simulink model "SegheriaSCADAdinamica"  (R2024b)
settings: Solver=FixedStepAuto  StartTime=0.0  StopTime=Tsim  FixedStep=dT  RelTol=1e-3
values from neighbouring files (symbols this model uses):
  b = t + 2*s    (= 3.6)    [ParametriSegheria.m]    (also in ParametriSegheriaDinamica.m)
  dT = 0.025    [ParametriSegheria.m]    (also in ParametriSegheriaDinamica.m)
  h_index = [70, 80, 90, 100]    [ParametriSegheria.m]    (also in ParametriSegheriaDinamica.m)
  J1 = 8*1e6    (= 8000000)    [ParametriSegheriaDinamica.m]
  J2 = 0.9*1e6    (= 900000)    [ParametriSegheriaDinamica.m]
  kc = [0 35 40 50 55 90]    [ParametriSegheria.m]    (also in ParametriSegheriaDinamica.m = [0, 25, 30, 35, 50, 70])
  Kt = 2    [ParametriSegheria.m]    (also in ParametriSegheriaDinamica.m = 10000)
  Kt2 = 5    [ParametriSegheria.m]    (also in ParametriSegheriaDinamica.m = 4500)
  l_index = [20, 30, 40, 50]    [ParametriSegheria.m]    (also in ParametriSegheriaDinamica.m)
  Lt = 4    [ParametriSegheria.m]    (also in ParametriSegheriaDinamica.m)
  Mag_D1 = [0 randi([220 500], 1, 40)]    [ParametriSegheria.m]    (also in ParametriSegheriaDinamica.m)
  Mag_D2 = [0 randi([220 500], 1, 40)]    [ParametriSegheria.m]    (also in ParametriSegheriaDinamica.m)
  Mag_D3 = [0 randi([220 500], 1, 40)]    [ParametriSegheria.m]    (also in ParametriSegheriaDinamica.m)
  Mag_legno1 = [0 randi([1 5], 1, 40)]    [ParametriSegheria.m]    (also in ParametriSegheriaDinamica.m)
  Mag_legno2 = [0 randi([1 5], 1, 40)]    [ParametriSegheria.m]    (also in ParametriSegheriaDinamica.m)
  Mag_legno3 = [0 randi([1 5], 1, 40)]    [ParametriSegheria.m]    (also in ParametriSegheriaDinamica.m)
  n_linee = 3    [ParametriSegheria.m]    (also in ParametriSegheriaDinamica.m)
  omega_ref1 = 50    [ParametriSegheriaDinamica.m]
  omega_ref2 = 3000*(2*pi/60)    (= 314.159265359)    [ParametriSegheriaDinamica.m]
  Rc = 200    [ParametriSegheria.m]    (also in ParametriSegheriaDinamica.m)
  rho = [0, 450, 520, 590, 710, 780]*1e-9    [ParametriSegheriaDinamica.m]
  Rs = 800    [ParametriSegheria.m]    (also in ParametriSegheriaDinamica.m)
  SR = Rs/Rm    (= 5.33333333333)    [ParametriSegheria.m]    (also in ParametriSegheriaDinamica.m)
  SR2 = Rc/Rm2    (= 4)    [ParametriSegheria.m]    (also in ParametriSegheriaDinamica.m)
  V_mean1 = 0.75    [ParametriSegheriaDinamica.m]
  V_mean23 = 1    [ParametriSegheriaDinamica.m]
undefined symbols (not defined in the file or in its folder): h_start_1, h_start_2, h_start_3, h_start_4, h_start_5, h_start_6, l_start_1, l_start_2, l_start_3, l_start_4, l_start_5, l_start_6
libraries: simulink x24, slpidlib x18
(part 4 of 4)

== matlab function SegheriaSCADAdinamica/Linea 2/MATLAB Function ==
  data: u input; y output
function y = fcn(u)

    persistent n_prec

    if isempty(n_prec)
        n_prec = 0;
    end

    y = u - n_prec;


    n_prec = u;

== matlab function SegheriaSCADAdinamica/Linea 2/MATLAB Function1 ==
  data: u input; y output
function y = fcn(u)

    persistent n_prec

    if isempty(n_prec)
        n_prec = 0;
    end

    y = u - n_prec;

    n_prec = u;

== matlab function SegheriaSCADAdinamica/Linea 2/MATLAB Function2 ==
  settings: updateMethod=DISCRETE
  data: lama_usurata input; y output; tronco_finito input
function y = fcn(lama_usurata, tronco_finito)
    
    persistent cambia_lama
    if isempty(cambia_lama)
        cambia_lama = 0;
    end

    if lama_usurata == 1
        cambia_lama = 1;
    end

    if tronco_finito == 1 && cambia_lama == 1
        y = cambia_lama;
        cambia_lama = 0;
    else
        y = 0;
    end

== matlab function SegheriaSCADAdinamica/Linea 2/MATLAB Function3 ==
  settings: updateMethod=DISCRETE
  data: u input; y output; t input
function y = f(u, t)
persistent t_start active

if isempty(active)
    active = false;
    t_start = 0;
end

if u == 1 && ~active
    t_start = t;
    active = true;
end

if active
    if (t - t_start) <= 180
        y = 0;
    else
        y = 1;
        active = false;
    end
else
    y = 1;
end

== matlab function SegheriaSCADAdinamica/Linea 2/Macchina 1/Dinamica Macchina 1/MATLAB Function3 ==
  data: w input; Fc output; vf input; kc input; Dt input; Rs parameter; b parameter
function Fc = Fcfun(w, vf, kc, Dt, Rs, b)

if w < 0.01
    Fc = 0;
else
    Fc = kc*b*vf*Dt/(w*Rs);
end

== matlab function SegheriaSCADAdinamica/Linea 2/Macchina 1/Logica Macchina 1/MATLAB Function ==
  data: u input; y output; Mag_legno parameter
function y = fcn(u, Mag_legno)
    persistent counter
    if isempty(counter)
        counter = 1;
    end

    if u == 1
        counter = counter + 1;
    end

    y = counter;
    
    if y > length(Mag_legno)-1
        y = 0;
    end

end

== matlab function SegheriaSCADAdinamica/Linea 3/MATLAB Function ==
  data: u input; y output
function y = fcn(u)

    persistent n_prec

    if isempty(n_prec)
        n_prec = 0;
    end

    y = u - n_prec;


    n_prec = u;

== matlab function SegheriaSCADAdinamica/Linea 3/MATLAB Function1 ==
  data: u input; y output
function y = fcn(u)

    persistent n_prec

    if isempty(n_prec)
        n_prec = 0;
    end

    y = u - n_prec;

    n_prec = u;

== matlab function SegheriaSCADAdinamica/Linea 3/MATLAB Function2 ==
  settings: updateMethod=DISCRETE
  data: lama_usurata input; y output; tronco_finito input
function y = fcn(lama_usurata, tronco_finito)
    
    persistent cambia_lama
    if isempty(cambia_lama)
        cambia_lama = 0;
    end

    if lama_usurata == 1
        cambia_lama = 1;
    end

    if tronco_finito == 1 && cambia_lama == 1
        y = cambia_lama;
        cambia_lama = 0;
    else
        y = 0;
    end

== matlab function SegheriaSCADAdinamica/Linea 3/MATLAB Function3 ==
  settings: updateMethod=DISCRETE
  data: u input; y output; t input
function y = f(u, t)
persistent t_start active

if isempty(active)
    active = false;
    t_start = 0;
end

if u == 1 && ~active
    t_start = t;
    active = true;
end

if active
    if (t - t_start) <= 180
        y = 0;
    else
        y = 1;
        active = false;
    end
else
    y = 1;
end

== matlab function SegheriaSCADAdinamica/Linea 3/Macchina 1/Dinamica Macchina 1/MATLAB Function3 ==
  data: w input; Fc output; vf input; kc input; Dt input; Rs parameter; b parameter
function Fc = Fcfun(w, vf, kc, Dt, Rs, b)

if w < 0.01
    Fc = 0;
else
    Fc = kc*b*vf*Dt/(w*Rs);
end

== matlab function SegheriaSCADAdinamica/Linea 1/Macchina 2/Dinamica Macchina 2/MATLAB Function3 ==
  data: w input; Fc output; vf input; kc input; ns input; h input; Rs parameter; b parameter
function Fc = Fcfun(w, vf, kc, ns, h, Rs, b)

if w < 0.01
    Fc = 0;
else
    Fc = ns*kc*b*vf*h/(w*Rs);
end

== matlab function SegheriaSCADAdinamica/Linea 3/Macchina 1/Logica Macchina 1/MATLAB Function ==
  data: u input; y output; Mag_legno parameter
function y = fcn(u, Mag_legno)
    persistent counter
    if isempty(counter)
        counter = 1;
    end

    if u == 1
        counter = counter + 1;
    end

    y = counter;
    
    if y > length(Mag_legno)-1
        y = 0;
    end

end

== matlab function SegheriaSCADAdinamica/Controllo Magazzino/MATLAB Function6 ==
  data: u input; idx output; h_index parameter
function idx = find_index(u, h_index)
%#codegen

v = h_index;

idx = -1; % valore default se non trovato

for i = 1:length(v)
    if u == v(i)
        idx = i;
        return;
    end
end

== matlab function SegheriaSCADAdinamica/Controllo Magazzino/MATLAB Function7 ==
  data: u input; idx output; h_index parameter
function idx = find_index(u, h_index)
%#codegen

v = h_index;

idx = -1; % valore default se non trovato

for i = 1:length(v)
    if u == v(i)
        idx = i;
        return;
    end
end

== matlab function SegheriaSCADAdinamica/Controllo Magazzino/MATLAB Function8 ==
  data: u input; idx output; h_index parameter
function idx = find_index(u, h_index)
%#codegen

v = h_index;

idx = -1; % valore default se non trovato

for i = 1:length(v)
    if u == v(i)
        idx = i;
        return;
    end
end

== matlab function SegheriaSCADAdinamica/Controllo Magazzino/MATLAB Function9 ==
  data: u input; idx output; h_index parameter
function idx = find_index(u, h_index)
%#codegen

v = h_index;

idx = -1; % valore default se non trovato

for i = 1:length(v)
    if u == v(i)
        idx = i;
        return;
    end
end

== matlab function SegheriaSCADAdinamica/Controllo Magazzino/MATLAB Function10 ==
  data: u input; idx output; l_index parameter
function idx = find_index(u, l_index)
%#codegen

v = l_index;

idx = -1; % valore default se non trovato

for i = 1:length(v)
    if u == v(i)
        idx = i;
        return;
    end
end

== matlab function SegheriaSCADAdinamica/Controllo Magazzino/MATLAB Function11 ==
  data: u input; idx output; l_index parameter
function idx = find_index(u, l_index)
%#codegen

v = l_index;

idx = -1; % valore default se non trovato

for i = 1:length(v)
    if u == v(i)
        idx = i;
        return;
    end
end

== matlab function SegheriaSCADAdinamica/Controllo Magazzino/MATLAB Function12 ==
  data: u input; idx output; l_index parameter
function idx = find_index(u, l_index)
%#codegen

v = l_index;

idx = -1; % valore default se non trovato

for i = 1:length(v)
    if u == v(i)
        idx = i;
        return;
    end
end

== matlab function SegheriaSCADAdinamica/Controllo Magazzino/MATLAB Function13 ==
  data: u input; idx output; l_index parameter
function idx = find_index(u, l_index)
%#codegen

v = l_index;

idx = -1; % valore default se non trovato

for i = 1:length(v)
    if u == v(i)
        idx = i;
        return;
    end
end

== matlab function SegheriaSCADAdinamica/Controllo Magazzino/MATLAB Function14 ==
  data: h_next output; Magazzino output; stop output; l_next output; h_idx input; target_matrice parameter; n_assi input; l_idx input
function [h_next, Magazzino, stop, l_next] = fcn(h_idx, target_matrice, n_assi, l_idx)

[n_rows, n_cols] = size(target_matrice);

h_next = zeros(1,length(h_idx));
l_next = zeros(1,length(l_idx));

persistent MagazzinoReale
persistent x_hat
persistent P


if isempty(MagazzinoReale)
    MagazzinoReale = zeros(n_rows, n_cols);
    x_hat = zeros(n_rows, n_cols);
    P = eye(n_rows*n_cols);
end

for i = 1:length(n_assi)

    % Output iniziali
    h_next(i) = h_idx(i);
    l_next(i) = l_idx(i);

    MagazzinoReale(h_idx(i), l_idx(i)) = MagazzinoReale(h_idx(i), l_idx(i)) + n_assi(i);

end
    
% MISURA RUMOROSA
sigma = 0.1;
y = MagazzinoReale + sigma*randn(size(MagazzinoReale));


% APPIATTISCO MATRICE
x_hat_vec = x_hat(:);
y_vec = y(:);
u = zeros(size(x_hat_vec));

% PREDICTION
Q = 0.01*eye(length(x_hat_vec));
x_pred = x_hat_vec + u;
P_pred = P + Q;

% UPDATE
R = 1*eye(length(x_hat_vec));
K = P_pred / (P_pred + R);
x_hat_vec = x_pred + K*(y_vec - x_pred);
P = (eye(size(K)) - K)*P_pred;

x_hat = reshape(x_hat_vec, n_rows, n_cols);


for i = 1:length(n_assi)
    if MagazzinoReale(h_idx(i), l_idx(i)) >= target_matrice(h_idx(i), l_idx(i))


        deficit = target_matrice - MagazzinoReale;

        best_cost = inf;
        best_h = h_idx(i);
        best_l = l_idx(i);

        for h = 1:n_rows
            for l = 1:n_cols

                if deficit(h,l) > 0

                    % Penalità cambio lama
                    cambio = (l ~= l_idx(i));

                    % Funzione costo
                    cost = -deficit(h,l) + 60*cambio;

                    if cost < best_cost
                        best_cost = cost;
                        best_h = h;
                        best_l = l;
                    end
                end

            end
        end

        if best_cost < inf
            h_next(i) = best_h;
            l_next(i) = best_l;
        end

    end
end

if MagazzinoReale >= target_matrice
    stop = 1;
else
    stop = 0;
end

Magazzino = MagazzinoReale;

== matlab function SegheriaSCADAdinamica/Linea 3/Macchina 1/Logica Macchina 1/MATLAB Function1 ==
  settings: updateMethod=DISCRETE
  data: spessore input; u input; spessore2 input; diametro input; y output; larg_asse output; thickness output; finito output; prior output; likelihood output; posterior output; larg_stim output
function [y, larg_asse, thickness, finito, prior, likelihood, posterior, larg_stim]= fcn(spessore, u, spessore2, diametro)
    persistent counter 
  
    thin_cut = 4;

    max_assi = floor((diametro-thin_cut*spessore2) / spessore);
    finito = 0;

    sigma_larg = 10;
    sigma_D = 10;

    if diametro > 0
        misure_D = diametro + sigma_D * randn();
    else
        misure_D = diametro;
    end

    maxD = 1000;
    larg_vec = 0:maxD;

    prior = zeros(size(larg_vec));
    likelihood = zeros(size(larg_vec));
    posterior = zeros(size(larg_vec));

    if isempty(counter)
        counter = 0;
    end

    % Conto assi tagliate
    if u == 1
        counter = counter + 1;
    end

    % Quando finisco tronco segnalo e azzero counter
    if counter > max_assi + thin_cut
        finito = 1;
        counter = 0;
    end

    % SISTEMARE INCERTEZZA: propagata da D in L
    if counter == 0
        larg_asse = 0;
        larg_asseD = 0;
        thickness = 0;
        sigma_largD = 0;
    elseif counter <= thin_cut/2
        distanza_bordo = counter * spessore2;
        larg_asse = sqrt((diametro)^2-(spessore2 + diametro - 2*distanza_bordo)^2);
        thickness = spessore2;
        % prior
        larg_asseD = sqrt(abs((misure_D)^2-(spessore2 + misure_D - 2*distanza_bordo)^2));
        sigma_largD = abs((2*distanza_bordo - spessore2)/sqrt((2*distanza_bordo - spessore2)*(-2*distanza_bordo + 2*diametro + spessore2)));
    elseif counter > max_assi + thin_cut/2
        distanza_bordo = max_assi*spessore + (counter-max_assi)*spessore2;
        larg_asse = sqrt((diametro)^2-(spessore2 + diametro - 2*distanza_bordo)^2);
        thickness = spessore2;
        % prior
        larg_asseD = sqrt(abs((misure_D)^2-(spessore2 + misure_D - 2*distanza_bordo)^2));
        sigma_largD = abs((2*distanza_bordo - spessore2)/sqrt((2*distanza_bordo - spessore2)*(-2*distanza_bordo + 2*diametro + spessore2)));
    else
        % Calcolo larghezza delle assi
        distanza_bordo = thin_cut/2 * spessore2 + (counter-thin_cut/2) * spessore;
        larg_asse = sqrt((diametro)^2-(spessore + diametro - 2*distanza_bordo)^2);
        thickness = spessore;
        % prior
        larg_asseD = sqrt(abs((misure_D)^2-(spessore2 + misure_D - 2*distanza_bordo)^2));
        sigma_largD = abs((2*distanza_bordo - spessore)/sqrt((2*distanza_bordo - spessore)*(-2*distanza_bordo + 2*diametro + spessore)));
    end

    if larg_asse > 0
        misure_larg = larg_asse + sigma_larg * randn();
    else
        misure_larg = larg_asse;
    end

    if larg_asse > 0
        prior(:) = 1/sqrt(2*pi*sigma_largD^2)*exp(-0.5 * ((larg_vec - larg_asseD) / sigma_largD).^2);
        prior(:) = prior(:) / sum(prior(:));
    else
        prior(:) = 0;
    end

    if misure_larg > 0
        likelihood(:) = 1/sqrt(2*pi*sigma_larg^2)*exp(-0.5 * ((larg_vec - misure_larg) / sigma_larg).^2);
        likelihood(:) = likelihood(:) / sum(likelihood(:));
    else
        likelihood(:) = 0;
    end

    if misure_larg > 0 && larg_asse > 0
        posterior(:) = prior(:) .* likelihood(:);
        posterior(:) = posterior(:) / sum(posterior(:));
    else
        posterior(:) = 0;
    end

    [~, idx] = max(posterior(:)); 

    larg_stim = larg_vec(idx);
    
    
    y = counter;

== matlab function SegheriaSCADAdinamica/Controllo Magazzino/CAMBIO LAME CONSUMATE ==
  data: n_assi input; y output; cambio_1 output; cambio_2 output; cambio_3 output; kc input; Lt parameter; b parameter; h input; lavoro_l output
function [y, cambio_1, cambio_2, cambio_3, lavoro_l] = fcn(n_assi, kc, Lt, b,h)

    warning = zeros(1, length(n_assi));

    persistent usura_lama
    persistent lavoro_lama

    if isempty(usura_lama)
        usura_lama = zeros(1, length(n_assi));
    end

    if isempty(lavoro_lama)
        lavoro_lama = zeros(1, length(n_assi));
    end

    cambio_1 = 0;
    cambio_2 = 0;
    cambio_3 = 0;

    for i = 1:length(n_assi)
        
        % Ogni volta che arriva un certo numero di assi vuol dire che le
        % lame hanno appena fatto un taglio
        if n_assi(i) ~= 0
            usura_lama(i) = usura_lama(i) + 1;
            lavoro_lama(i) = lavoro_lama(i) + kc(i)*b*Lt*h(i);
        end
        
        if lavoro_lama(i) > 600000
            warning(i) = 1;
            lavoro_lama(i) = 0;
        end

        % i = 1 -> M2 Linea 1
        % i = 2 -> M3 Linea 1
        % i = 3 -> M2 Linea 2
        % i = 4 -> M3 Linea 2
        % i = 5 -> M2 Linea 3
        % i = 6 -> M2 Linea 3
        if (i == 1 || i == 2) && warning(i) == 1
            cambio_1 = 1;
        elseif (i == 3 || i == 4) && warning(i) == 1
            cambio_2 = 1;
        elseif (i == 5 || i == 6) && warning(i) == 1
            cambio_3 = 1;
        end

    end

    lavoro_l = lavoro_lama;

    y = warning;

== matlab function SegheriaSCADAdinamica/Linea 1/MATLAB Function3 ==
  settings: updateMethod=DISCRETE
  data: u input; y output; t input
function y = f(u, t)
persistent t_start active

if isempty(active)
    active = false;
    t_start = 0;
end

if u == 1 && ~active
    t_start = t;
    active = true;
end

if active
    if (t - t_start) <= 180
        y = 0;
    else
        y = 1;
        active = false;
    end
else
    y = 1;
end

== matlab function SegheriaSCADAdinamica/Linea 2/Macchina 2/Dinamica Macchina 2/MATLAB Function3 ==
  data: w input; Fc output; vf input; kc input; ns input; h input; Rs parameter; b parameter
function Fc = Fcfun(w, vf, kc, ns, h, Rs, b)

if w < 0.01
    Fc = 0;
else
    Fc = ns*kc*b*vf*h/(w*Rs);
end

== matlab function SegheriaSCADAdinamica/Linea 1/Macchina 1/Logica Macchina 1/MATLAB Function ==
  data: u input; y output; Mag_legno parameter
function y = fcn(u, Mag_legno)
    persistent counter
    if isempty(counter)
        counter = 1;
    end

    if u == 1
        counter = counter + 1;
    end

    y = counter;
    
    if y > length(Mag_legno)-1
        y = 0;
    end

end

== matlab function SegheriaSCADAdinamica/Linea 1/Macchina 2/MATLAB Function2 ==
  settings: updateMethod=DISCRETE
  data: u input; w_asse input; y output; l_asse input; taglio output; Lt parameter
function [y, taglio] = fcn(u, w_asse, l_asse,Lt)
    persistent counter 

    n_assi = floor(l_asse / w_asse);
    
    taglio = 0;

    if isempty(counter)
        counter = 0;
    end

    % Conto assi tagliate
    if u >= Lt
        counter = counter + n_assi;
    end

    % Segnale di taglio
    if  (u > 0 && u < Lt && l_asse > 0) 
        taglio = 1;
    end
    y = counter;
end

== matlab function SegheriaSCADAdinamica/Linea 3/Macchina 2/Dinamica Macchina 2/MATLAB Function3 ==
  data: w input; Fc output; vf input; kc input; ns input; h input; Rs parameter; b parameter
function Fc = Fcfun(w, vf, kc, ns, h, Rs, b)

if w < 0.01
    Fc = 0;
else
    Fc = ns*kc*b*vf*h/(w*Rs);
end

== matlab function SegheriaSCADAdinamica/Linea 1/Macchina 3/Dinamica Macchina 2/MATLAB Function3 ==
  data: w input; Fc output; vf input; kc input; ns input; h input; Rs parameter; b parameter
function Fc = Fcfun(w, vf, kc, ns, h, Rs, b)

if w < 0.01
    Fc = 0;
else
    Fc = ns*kc*b*vf*h/(w*Rs);
end

== matlab function SegheriaSCADAdinamica/Linea 1/Macchina 3/MATLAB Function2 ==
  settings: updateMethod=DISCRETE
  data: u input; w_asse input; y output; l_asse input; taglio output; Lt parameter
function [y, taglio] = fcn(u, w_asse, l_asse,Lt)
    persistent counter 

    n_assi = floor(l_asse / w_asse);
    
    taglio = 0;

    if isempty(counter)
        counter = 0;
    end

    % Conto assi tagliate
    if u >= Lt
        counter = counter + n_assi;
    end

    % Segnale di taglio
    if  (u > 0 && u < Lt && l_asse > 0) 
        taglio = 1;
    end
    y = counter;
end

== matlab function SegheriaSCADAdinamica/Linea 1/MATLAB Function2 ==
  settings: updateMethod=DISCRETE
  data: lama_usurata input; y output; tronco_finito input
function y = fcn(lama_usurata, tronco_finito)
    
    persistent cambia_lama
    if isempty(cambia_lama)
        cambia_lama = 0;
    end

    if lama_usurata == 1
        cambia_lama = 1;
    end

    if tronco_finito == 1 && cambia_lama == 1
        y = cambia_lama;
        cambia_lama = 0;
    else
        y = 0;
    end

== matlab function SegheriaSCADAdinamica/Linea 2/Macchina 2/MATLAB Function2 ==
  settings: updateMethod=DISCRETE
  data: u input; w_asse input; y output; l_asse input; taglio output; Lt parameter
function [y, taglio] = fcn(u, w_asse, l_asse,Lt)
    persistent counter 

    n_assi = floor(l_asse / w_asse);
    
    taglio = 0;

    if isempty(counter)
        counter = 0;
    end

    % Conto assi tagliate
    if u >= Lt
        counter = counter + n_assi;
    end

    % Segnale di taglio
    if  (u > 0 && u < Lt && l_asse > 0) 
        taglio = 1;
    end
    y = counter;
end

== matlab function SegheriaSCADAdinamica/Linea 2/Macchina 3/Dinamica Macchina 2/MATLAB Function3 ==
  data: w input; Fc output; vf input; kc input; ns input; h input; Rs parameter; b parameter
function Fc = Fcfun(w, vf, kc, ns, h, Rs, b)

if w < 0.01
    Fc = 0;
else
    Fc = ns*kc*b*vf*h/(w*Rs);
end

== matlab function SegheriaSCADAdinamica/Linea 1/Macchina 1/Logica Macchina 1/MATLAB Function2 ==
  settings: updateMethod=DISCRETE
  data: spessore input; u input; spessore2 input; diametro input; y output; larg_asse output; thickness output; finito output; prior output; likelihood output; posterior output; larg_stim output
function [y, larg_asse, thickness, finito, prior, likelihood, posterior, larg_stim]= fcn(spessore, u, spessore2, diametro)
    persistent counter 
  
    thin_cut = 4;

    max_assi = floor((diametro-thin_cut*spessore2) / spessore);
    finito = 0;

    sigma_larg = 10;
    sigma_D = 10;

    if diametro > 0
        misure_D = diametro + sigma_D * randn();
    else
        misure_D = diametro;
    end

    maxD = 1000;
    larg_vec = 0:maxD;

    prior = zeros(size(larg_vec));
    likelihood = zeros(size(larg_vec));
    posterior = zeros(size(larg_vec));

    if isempty(counter)
        counter = 0;
    end

    % Conto assi tagliate
    if u == 1
        counter = counter + 1;
    end

    % Quando finisco tronco segnalo e azzero counter
    if counter > max_assi + thin_cut
        finito = 1;
        counter = 0;
    end

    % SISTEMARE INCERTEZZA: propagata da D in L
    if counter == 0
        larg_asse = 0;
        larg_asseD = 0;
        thickness = 0;
        sigma_largD = 0;
    elseif counter <= thin_cut/2
        distanza_bordo = counter * spessore2;
        larg_asse = sqrt((diametro)^2-(spessore2 + diametro - 2*distanza_bordo)^2);
        thickness = spessore2;
        % prior
        larg_asseD = sqrt(abs((misure_D)^2-(spessore2 + misure_D - 2*distanza_bordo)^2));
        sigma_largD = abs((2*distanza_bordo - spessore2)/sqrt((2*distanza_bordo - spessore2)*(-2*distanza_bordo + 2*diametro + spessore2)));
    elseif counter > max_assi + thin_cut/2
        distanza_bordo = max_assi*spessore + (counter-max_assi)*spessore2;
        larg_asse = sqrt((diametro)^2-(spessore2 + diametro - 2*distanza_bordo)^2);
        thickness = spessore2;
        % prior
        larg_asseD = sqrt(abs((misure_D)^2-(spessore2 + misure_D - 2*distanza_bordo)^2));
        sigma_largD = abs((2*distanza_bordo - spessore2)/sqrt((2*distanza_bordo - spessore2)*(-2*distanza_bordo + 2*diametro + spessore2)));
    else
        % Calcolo larghezza delle assi
        distanza_bordo = thin_cut/2 * spessore2 + (counter-thin_cut/2) * spessore;
        larg_asse = sqrt((diametro)^2-(spessore + diametro - 2*distanza_bordo)^2);
        thickness = spessore;
        % prior
        larg_asseD = sqrt(abs((misure_D)^2-(spessore2 + misure_D - 2*distanza_bordo)^2));
        sigma_largD = abs((2*distanza_bordo - spessore)/sqrt((2*distanza_bordo - spessore)*(-2*distanza_bordo + 2*diametro + spessore)));
    end

    if larg_asse > 0
        misure_larg = larg_asse + sigma_larg * randn();
    else
        misure_larg = larg_asse;
    end

    if larg_asse > 0
        prior(:) = 1/sqrt(2*pi*sigma_largD^2)*exp(-0.5 * ((larg_vec - larg_asseD) / sigma_largD).^2);
        prior(:) = prior(:) / sum(prior(:));
    else
        prior(:) = 0;
    end

    if misure_larg > 0
        likelihood(:) = 1/sqrt(2*pi*sigma_larg^2)*exp(-0.5 * ((larg_vec - misure_larg) / sigma_larg).^2);
        likelihood(:) = likelihood(:) / sum(likelihood(:));
    else
        likelihood(:) = 0;
    end

    if misure_larg > 0 && larg_asse > 0
        posterior(:) = prior(:) .* likelihood(:);
        posterior(:) = posterior(:) / sum(posterior(:));
    else
        posterior(:) = 0;
    end

    [~, idx] = max(posterior(:)); 

    larg_stim = larg_vec(idx);
    
    
    y = counter;

== matlab function SegheriaSCADAdinamica/Linea 2/Macchina 3/MATLAB Function2 ==
  settings: updateMethod=DISCRETE
  data: u input; w_asse input; y output; l_asse input; taglio output; Lt parameter
function [y, taglio] = fcn(u, w_asse, l_asse,Lt)
    persistent counter 

    n_assi = floor(l_asse / w_asse);
    
    taglio = 0;

    if isempty(counter)
        counter = 0;
    end

    % Conto assi tagliate
    if u >= Lt
        counter = counter + n_assi;
    end

    % Segnale di taglio
    if  (u > 0 && u < Lt && l_asse > 0) 
        taglio = 1;
    end
    y = counter;
end

== matlab function SegheriaSCADAdinamica/Linea 3/Macchina 2/MATLAB Function2 ==
  settings: updateMethod=DISCRETE
  data: u input; w_asse input; y output; l_asse input; taglio output; Lt parameter
function [y, taglio] = fcn(u, w_asse, l_asse,Lt)
    persistent counter 

    n_assi = floor(l_asse / w_asse);
    
    taglio = 0;

    if isempty(counter)
        counter = 0;
    end

    % Conto assi tagliate
    if u >= Lt
        counter = counter + n_assi;
    end

    % Segnale di taglio
    if  (u > 0 && u < Lt && l_asse > 0) 
        taglio = 1;
    end
    y = counter;
end

== matlab function SegheriaSCADAdinamica/Linea 3/Macchina 3/Dinamica Macchina 2/MATLAB Function3 ==
  data: w input; Fc output; vf input; kc input; ns input; h input; Rs parameter; b parameter
function Fc = Fcfun(w, vf, kc, ns, h, Rs, b)

if w < 0.01
    Fc = 0;
else
    Fc = ns*kc*b*vf*h/(w*Rs);
end

== matlab function SegheriaSCADAdinamica/Linea 3/Macchina 3/MATLAB Function2 ==
  settings: updateMethod=DISCRETE
  data: u input; w_asse input; y output; l_asse input; taglio output; Lt parameter
function [y, taglio] = fcn(u, w_asse, l_asse,Lt)
    persistent counter 

    n_assi = floor(l_asse / w_asse);
    
    taglio = 0;

    if isempty(counter)
        counter = 0;
    end

    % Conto assi tagliate
    if u >= Lt
        counter = counter + n_assi;
    end

    % Segnale di taglio
    if  (u > 0 && u < Lt && l_asse > 0) 
        taglio = 1;
    end
    y = counter;
end

== matlab function SegheriaSCADAdinamica/MATLAB Function ==
  data: v_ref1 output; v_ref23 output; n_attive input; n_linee parameter; V_mean1 parameter; V_mean23 parameter
function [v_ref1,v_ref23] = fcn(n_attive, n_linee, V_mean1, V_mean23)

if n_attive == 0
    v_ref1 = 0.01;
    v_ref23 = 0.01;
else
    v_ref1 = n_linee*V_mean1/n_attive;
    v_ref23 = n_linee*V_mean23/n_attive;
end

== matlab function SegheriaSCADAdinamica/Controllo Magazzino/MATLAB Function ==
  data: true_n_assi input; n_assi_estimate output; true_larg input; width_cut input; t2 parameter; posterior output; likelihood output; prior output
function [n_assi_estimate, posterior, likelihood, prior]= fcn(true_n_assi, true_larg, width_cut, t2)

    n_assi_estimate = zeros(1, length(true_n_assi));
    
    
    % persistent step_counter
    

    % if isempty(step_counter)
    %     step_counter = 0;
    % end

    sigma_larg = 50;     % Uncertainty (mm)
    sigma_cam = 0.5;    % Uncertainty of the camera
    max_N = 30;         % Max boards number

    misure_larg = true_larg + sigma_larg * randn();
    misure_camera = true_n_assi + sigma_cam * randn();

    posterior = zeros(max_N, length(true_n_assi));
    likelihood = zeros(max_N, length(true_n_assi));
    prior = zeros(max_N, length(true_n_assi));

    for i = 1:length(true_n_assi)

        n_vec = 1:max_N;

        if true_n_assi(i) ~= 0
        
            % Compute the prior (probability distribution for each board number
            % given that measure)
            % mu_larg = n_vec * width_cut(i); % + ((n_vec - 1) * t2);
            % prior(:, i) = exp(-0.5 * ((misure_larg(i) - mu_larg) / sigma_larg).^2);

            sigma_nl = sigma_larg/width_cut(i);
            n_larg = floor(misure_larg(i)/width_cut(i));
            
            prior(:, i) = 1/sqrt(2*pi*sigma_nl^2)*exp(-0.5 * ((n_vec - n_larg) / sigma_nl).^2);
            prior(:, i) = prior(:, i) / sum(prior(:, i));

            % Compute the likelihood from the camera sensor
            likelihood(:, i) = 1/sqrt(2*pi*sigma_cam^2)*exp(-0.5 * ((n_vec - misure_camera(i)) / sigma_cam).^2);
            likelihood(:, i) = likelihood(:, i) / sum(likelihood(:, i));
        

            % Compute the posterior - Bayesyan fusion
            % Riempio posteriori per ogni macchina così posso plottare la
            % distribuzione
            posterior(:, i) = prior(:, i) .* likelihood(:, i);
            posterior(:, i) = posterior(:, i) / sum(posterior(:, i));
            [~, idx] = max(posterior(:, i)); % MAP 

            n_assi_estimate(i) = n_vec(idx);
        else
            n_assi_estimate(i) = 0;
        end
    end


 % step_counter = step_counter + 1;

== matlab function SegheriaSCADAdinamica/Controllo Magazzino/MATLAB Function15 ==
  data: true_n_assi input; n_assi_estimate output; true_larg input; width_cut input
function n_assi_estimate= fcn(true_n_assi, true_larg, width_cut)

    
    persistent stima_n

    if isempty(stima_n)
        stima_n = 0;
    end


    sigma_larg = 2;     % Uncertainty (mm)
    sigma_cam = 1;      % Uncertainty of the camera
    max_N = 50;         % Max boards number

    
    if true_n_assi(1) ~= 0
        
        n_vec = 1:max_N;
    
        % Compute the prior (probability distribution for each board number
        % given that measure)
        mu_larg = n_vec * width_cut;
        prior = exp(-0.5 * ((true_larg - mu_larg) / sigma_larg).^2);
        prior = prior / sum(prior);

        % Compute the likelihood from the camera sensor
        likelihood = exp(-0.5 * ((n_vec - true_n_assi(1)) / sigma_cam).^2);
        likelihood = likelihood / sum(likelihood);
        

        % Compute the posterior - Bayesyan fusion
        posterior = prior .* likelihood;
        [~, idx] = max(posterior); % MAP 

        n_assi_estimate = n_vec(idx);

    else
        n_assi_estimate = 0;
    end

== matlab function SegheriaSCADAdinamica/Linea 2/Macchina 1/Logica Macchina 1/MATLAB Function1 ==
  settings: updateMethod=DISCRETE
  data: spessore input; u input; spessore2 input; diametro input; y output; larg_asse output; thickness output; finito output; prior output; likelihood output; posterior output; larg_stim output
function [y, larg_asse, thickness, finito, prior, likelihood, posterior, larg_stim]= fcn(spessore, u, spessore2, diametro)
    persistent counter 
  
    thin_cut = 4;

    max_assi = floor((diametro-thin_cut*spessore2) / spessore);
    finito = 0;

    sigma_larg = 10;
    sigma_D = 10;

    if diametro > 0
        misure_D = diametro + sigma_D * randn();
    else
        misure_D = diametro;
    end

    maxD = 1000;
    larg_vec = 0:maxD;

    prior = zeros(size(larg_vec));
    likelihood = zeros(size(larg_vec));
    posterior = zeros(size(larg_vec));

    if isempty(counter)
        counter = 0;
    end

    % Conto assi tagliate
    if u == 1
        counter = counter + 1;
    end

    % Quando finisco tronco segnalo e azzero counter
    if counter > max_assi + thin_cut
        finito = 1;
        counter = 0;
    end

    % SISTEMARE INCERTEZZA: propagata da D in L
    if counter == 0
        larg_asse = 0;
        larg_asseD = 0;
        thickness = 0;
        sigma_largD = 0;
    elseif counter <= thin_cut/2
        distanza_bordo = counter * spessore2;
        larg_asse = sqrt((diametro)^2-(spessore2 + diametro - 2*distanza_bordo)^2);
        thickness = spessore2;
        % prior
        larg_asseD = sqrt(abs((misure_D)^2-(spessore2 + misure_D - 2*distanza_bordo)^2));
        sigma_largD = abs((2*distanza_bordo - spessore2)/sqrt((2*distanza_bordo - spessore2)*(-2*distanza_bordo + 2*diametro + spessore2)));
    elseif counter > max_assi + thin_cut/2
        distanza_bordo = max_assi*spessore + (counter-max_assi)*spessore2;
        larg_asse = sqrt((diametro)^2-(spessore2 + diametro - 2*distanza_bordo)^2);
        thickness = spessore2;
        % prior
        larg_asseD = sqrt(abs((misure_D)^2-(spessore2 + misure_D - 2*distanza_bordo)^2));
        sigma_largD = abs((2*distanza_bordo - spessore2)/sqrt((2*distanza_bordo - spessore2)*(-2*distanza_bordo + 2*diametro + spessore2)));
    else
        % Calcolo larghezza delle assi
        distanza_bordo = thin_cut/2 * spessore2 + (counter-thin_cut/2) * spessore;
        larg_asse = sqrt((diametro)^2-(spessore + diametro - 2*distanza_bordo)^2);
        thickness = spessore;
        % prior
        larg_asseD = sqrt(abs((misure_D)^2-(spessore2 + misure_D - 2*distanza_bordo)^2));
        sigma_largD = abs((2*distanza_bordo - spessore)/sqrt((2*distanza_bordo - spessore)*(-2*distanza_bordo + 2*diametro + spessore)));
    end

    if larg_asse > 0
        misure_larg = larg_asse + sigma_larg * randn();
    else
        misure_larg = larg_asse;
    end

    if larg_asse > 0
        prior(:) = 1/sqrt(2*pi*sigma_largD^2)*exp(-0.5 * ((larg_vec - larg_asseD) / sigma_largD).^2);
        prior(:) = prior(:) / sum(prior(:));
    else
        prior(:) = 0;
    end

    if misure_larg > 0
        likelihood(:) = 1/sqrt(2*pi*sigma_larg^2)*exp(-0.5 * ((larg_vec - misure_larg) / sigma_larg).^2);
        likelihood(:) = likelihood(:) / sum(likelihood(:));
    else
        likelihood(:) = 0;
    end

    if misure_larg > 0 && larg_asse > 0
        posterior(:) = prior(:) .* likelihood(:);
        posterior(:) = posterior(:) / sum(posterior(:));
    else
        posterior(:) = 0;
    end

    [~, idx] = max(posterior(:)); 

    larg_stim = larg_vec(idx);
    
    
    y = counter;

== matlab function SegheriaSCADAdinamica/Linea 1/Macchina 1/Dinamica Macchina 1/MATLAB Function3 ==
  data: w input; Fc output; vf input; kc input; Dt input; Rs parameter; b parameter
function Fc = Fcfun(w, vf, kc, Dt, Rs, b)

if w < 0.01
    Fc = 0;
else
    Fc = kc*b*vf*Dt/(w*Rs);
end

== matlab function SegheriaSCADAdinamica/Linea 1/MATLAB Function ==
  data: u input; y output
function y = fcn(u)

    persistent n_prec

    if isempty(n_prec)
        n_prec = 0;
    end

    y = u - n_prec;


    n_prec = u;

== matlab function SegheriaSCADAdinamica/Controllo Magazzino/MATLAB Function1 ==
  data: u input; idx output; h_index parameter
function idx = find_index(u, h_index)
%#codegen

v = h_index;

idx = -1; % valore default se non trovato

for i = 1:length(v)
    if u == v(i)
        idx = i;
        return;
    end
end

== matlab function SegheriaSCADAdinamica/Controllo Magazzino/MATLAB Function2 ==
  data: u input; idx output; l_index parameter
function idx = find_index(u, l_index)
%#codegen

v = l_index;

idx = -1; % valore default se non trovato

for i = 1:length(v)
    if u == v(i)
        idx = i;
        return;
    end
end

== matlab function SegheriaSCADAdinamica/Controllo Magazzino/MATLAB Function3 ==
  data: h_next output; Magazzino output; stop output; l_next output; h_idx input; target_matrice parameter; n_assi input; l_idx input
function [h_next, Magazzino, stop, l_next] = fcn(h_idx, target_matrice, n_assi, l_idx)

[n_rows, n_cols] = size(target_matrice);

h_next = zeros(1,length(h_idx));
l_next = zeros(1,length(l_idx));

persistent MagazzinoReale




if isempty(MagazzinoReale)
    MagazzinoReale = zeros(n_rows, n_cols);
end

for i = 1:length(n_assi)
    % Output iniziali
    h_next(i) = h_idx(i);
    l_next(i) = l_idx(i);

    MagazzinoReale(h_idx(i), l_idx(i)) = MagazzinoReale(h_idx(i), l_idx(i)) + n_assi(i);
end
    


for i = 1:length(n_assi)
    if MagazzinoReale(h_idx(i), l_idx(i)) >= target_matrice(h_idx(i), l_idx(i))


        deficit = target_matrice - MagazzinoReale;

        best_cost = inf;
        best_h = h_idx(i);
        best_l = l_idx(i);

        for h = 1:n_rows
            for l = 1:n_cols

                if deficit(h,l) > 0

                    % Penalità cambio lama
                    cambio = (l ~= l_idx(i));

                    % Funzione costo
                    cost = -deficit(h,l) + 60*cambio;

                    if cost < best_cost
                        best_cost = cost;
                        best_h = h;
                        best_l = l;
                    end
                end

            end
        end

        if best_cost < inf
            h_next(i) = best_h;
            l_next(i) = best_l;
        end

    end
end

if MagazzinoReale >= target_matrice
    stop = 1;
else
    stop = 0;
end

Magazzino = MagazzinoReale;
